simulink model "MotorModel_3"  (R2018b)
settings: Solver=VariableStepDiscrete  StartTime=0.0  StopTime=6  RelTol=1e-3  EnableMultiTasking=on
libraries: powerlib x22, powerlib_meascontrol x3, simulink x1
settings Model: Creator=LXQ  LastModifiedBy=Administrator
settings SolverCC: ZeroCrossControl=DisableAll
settings DataIOCC: LimitDataPoints=on  SaveFormat=Array
settings OptimizationCC: LifeSpan=inf
settings DebuggingCC: SolverPrmCheckMsg=warning  SFUnexpectedBacktrackingDiag=warning  SFNoUnconditionalDefaultTransitionDiag=warning  SFExecutionAtInitializationDiag=none
settings HardwareCC: ProdBitPerPointer=32  ProdBitPerSizeT=32  ProdBitPerPtrDiffT=32  ProdLargestAtomicFloat=None  ProdIntDivRoundTo=Undefined  ProdEndianess=Unspecified  ProdWordSize=32  ProdHWDeviceType=32-bit Generic
settings ModelReferenceCC: PropagateSignalLabelsOutOfModel=off
settings SFSimCC: SimUseLocalCustomCode=off
settings RTWCC: RTWUseLocalCustomCode=off
settings CodeAppCC: StateflowObjectComments=on
settings GRTTargetCC: TargetLangStandard=C89/C90 (ANSI)  GeneratePreprocessorConditionals=Disable all
settings ConfigComp: CovMetricSettings=dw  CovHtmlReporting=on  CovSaveCumulativeToWorkspaceVar=on  CovSaveSingleToWorkspaceVar=on  CovExternalEMLEnable=off  CovSFcnEnable=off
settings SimscapeCC: SimscapeNormalizeSystem=off

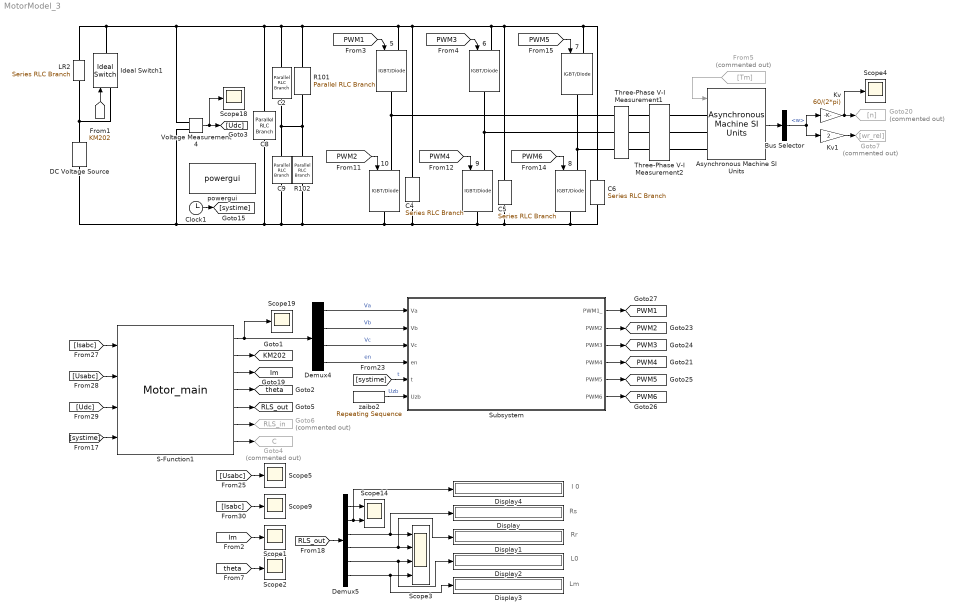
== system MotorModel_3 ==
  note: Rs
  note: Rr
  note: L0
  note: Lm
  note: I 0
  {5..10} (6 alike) : powerlib/Power Electronics/IGBT//Diode  Ron=1e-3  Rs=5000  Cs=inf  Measurements=off
      settings: SourceProductName=Simscape Electrical
  Asynchronous Machine SI Units : powerlib/Machines/Asynchronous Machine SI Units  RotorType=Squirrel-cage  PresetModel=No  MechanicalLoad=Torque Tm  ShowDetailedParameters=on  ReferenceFrame=Synchronous  Units=SI  MeasurementBus=on  NominalParameters=[41000 220 50]  Stator=[0.048 0.00031]  Rotor=[0.019 0.00031]  Cage1=[ 0.022 0.226/377]  Cage2=[ 0.022 0.226/377]  Lm=0.0133  Mechanical=[0.4 0.02187 2]  PolePairs=2  InitialConditions=[1 0 0 0 0 0 0 0]  SimulateSaturation=off  Saturation=[14.03593122, 27.81365428, 53.79336849, 72.68890987, 97.98006896, 148.6815601, 215.7428561, 302.9841135, 420.4778367 ; 230, 322, 414, 460, 506, 552, 598, 644, 690]  LoadFlowParameters=1492000  TsPowergui=0  TsBlock=-1  IterativeModel=Trapezoidal non iterative  IterativeDiscreteModel=Trapezoidal non iterative  Pmec=0
      settings: SourceProductName=Simscape Electrical
  Bus Selector : BusSelector  OutputSignals=w
  C2 : powerlib/Elements/Parallel RLC Branch  LConnTagsString=a  RConnTagsString=__new0  BranchType=C  Resistance=1  Inductance=1e-3  SetiL0=off  InitialCurrent=0  Capacitance=400e-6  Setx0=off  InitialVoltage=0  Measurements=None
      settings: SourceProductName=Simscape Electrical
  C4 : powerlib/Elements/Series RLC Branch  LConnTagsString=__new0  RConnTagsString=__new0  BranchType=C  Resistance=10  Inductance=40e-9  SetiL0=off  InitialCurrent=0  Capacitance=0.47e-6  Setx0=off  InitialVoltage=0  Measurements=None
      settings: SourceProductName=Simscape Electrical
  C5 : powerlib/Elements/Series RLC Branch  LConnTagsString=__new0  RConnTagsString=__new0  BranchType=C  Resistance=10  Inductance=40e-9  SetiL0=off  InitialCurrent=0  Capacitance=0.47e-6  Setx0=off  InitialVoltage=0  Measurements=None
      settings: SourceProductName=Simscape Electrical
  C6 : powerlib/Elements/Series RLC Branch  LConnTagsString=__new0  RConnTagsString=__new0  BranchType=C  Resistance=10  Inductance=40e-9  SetiL0=off  InitialCurrent=0  Capacitance=0.47e-6  Setx0=off  InitialVoltage=0  Measurements=None
      settings: SourceProductName=Simscape Electrical
  C8 : powerlib/Elements/Parallel RLC Branch  LConnTagsString=a  RConnTagsString=__new0  BranchType=C  Resistance=15e3  Inductance=1e-3  SetiL0=off  InitialCurrent=0  Capacitance=400e-6  Setx0=off  InitialVoltage=0  Measurements=None
      settings: SourceProductName=Simscape Electrical
  C9 : powerlib/Elements/Parallel RLC Branch  LConnTagsString=a  RConnTagsString=__new0  BranchType=C  Resistance=1  Inductance=1e-3  SetiL0=off  InitialCurrent=0  Capacitance=400e-6  Setx0=off  InitialVoltage=0  Measurements=None
      settings: SourceProductName=Simscape Electrical
  Clock1 : Clock
  DC Voltage Source : powerlib/Electrical Sources/DC Voltage Source  Amplitude=470  Measurements=None
      settings: SourceProductName=Simscape Electrical
  Demux4 : Demux
  Demux5 : Demux  Outputs=6
  Display{,1..4} (5 alike) : Display
  From5 : From  Commented=on  GotoTag=Tm
  Goto20 : Goto  Commented=on  GotoTag=n
  Goto4 : Goto  Commented=on  GotoTag=C  TagVisibility=global
  Goto6 : Goto  Commented=on  GotoTag=RLS_in  TagVisibility=global
  Goto7 : Goto  Commented=on  GotoTag=wr_rel
  Ideal Switch1 : powerlib/Power Electronics/Ideal Switch  Ron=0.0000000001  Lon=0  IC=0  Rs=1e7  Cs=inf  Measurements=off
      settings: SourceProductName=Simscape Electrical
  Kv : Gain  Gain=60/(2*pi)  SaturateOnIntegerOverflow=on  OutDataTypeStr=Inherit: Same as input  ParamDataTypeStr=Inherit: Same as input
  Kv1 : Gain  Gain=2  SaturateOnIntegerOverflow=on  OutDataTypeStr=Inherit: Same as input  ParamDataTypeStr=Inherit: Same as input
  LR2 : powerlib/Elements/Series RLC Branch  LConnTagsString=__new0  RConnTagsString=__new0  BranchType=R  Resistance=30  Inductance=200e-6  SetiL0=off  InitialCurrent=0  Capacitance=1e-6  Setx0=off  InitialVoltage=0  Measurements=None
      settings: SourceProductName=Simscape Electrical
  R101 : powerlib/Elements/Parallel RLC Branch  LConnTagsString=a  RConnTagsString=__new0  BranchType=R  Resistance=15e3  Inductance=1e-3  SetiL0=off  InitialCurrent=0  Capacitance=10800e-6  Setx0=on  InitialVoltage=110  Measurements=None
      settings: SourceProductName=Simscape Electrical
  R102 : powerlib/Elements/Parallel RLC Branch  LConnTagsString=a  RConnTagsString=__new0  BranchType=R  Resistance=15e3  Inductance=1e-3  SetiL0=off  InitialCurrent=0  Capacitance=10800e-6  Setx0=on  InitialVoltage=110  Measurements=None
      settings: SourceProductName=Simscape Electrical
  S-Function1 : S-Function  FunctionName=Motor_main  SFunctionDeploymentMode=off  EnableBusSupport=off
  Scope{1..2,4..5,9,18..19} (7 alike) : Scope
  Scope14 : Scope  NumInputPorts=2
  Scope3 : Scope  NumInputPorts=4
  Subsystem : Subsystem
  Three-Phase V-I Measurement1 : powerlib/Measurements/Three-Phase V-I Measurement  VoltageMeasurement=phase-to-phase  SetLabelV=on  LabelV=Uabc  Vpu=off  VpuLL=off  CurrentMeasurement=yes  SetLabelI=on  LabelI=Isabc  Ipu=off  Pbase=100e6  Vbase=500e3  OutputType=Complex  PhasorSimulation=off  PSBequivalent=0
      settings: SourceProductName=Simscape Electrical
  Three-Phase V-I Measurement2 : powerlib/Measurements/Three-Phase V-I Measurement  VoltageMeasurement=phase-to-phase  SetLabelV=on  LabelV=Usabc  Vpu=off  VpuLL=off  CurrentMeasurement=yes  SetLabelI=on  LabelI=Iabc  Ipu=off  Pbase=100e6  Vbase=500e3  OutputType=Complex  PhasorSimulation=off  PSBequivalent=0
      settings: SourceProductName=Simscape Electrical
  Voltage Measurement4 : powerlib/Measurements/Voltage Measurement  PhasorSimulation=off  OutputType=Complex  PSBequivalent=0
      settings: SourceProductName=Simscape Electrical
  powergui : powerlib/powergui  Priority=1  SimulationMode=Discrete  SampleTime=0.5e-6  frequency=60  Iterations=50  frequencyindice=0  Pbase=100e6  ErrMax=1e-4  UnitsV=kV  UnitsW=MW  buscounter=0  FunctionMessages=off  echomessages=off  EnableUseOfTLC=off  CurrentSourceSwitches=off  DisableSnubberDevices=off  DisableRonSwitches=off  DisableVfSwitches=off  DisplayEquations=off  SolverType=Tustin  Interpol=off  ExternalGateDelay=off  methode=off  Ts=0  x0status=blocks  SPID=off  SwTol=0  HookPort=off  RestoreLinks=warning  ResistiveCurrentMeasurement=off  Frange=[0:2:500]  Ylog=off  Xlog=on  ShowGrid=off  save=off  variable=ZData  structure=0  ZoomFFT=off  StartTime=0.0  cycles=1  DisplayStyle=1  fundamental=60  FreqAxis=off  MaxFrequency=1000  frequencyindicesteady=1  RmsSteady=1  display=off
      settings: SourceProductName=Simscape Electrical
  zaibo2 : simulink/Sources/Repeating Sequence  rep_seq_t=[0 1/10000 1/5000]  rep_seq_y=[-1 1 -1]
  tag scope: Im=global, KM202=global, PWM1=global, PWM2=global, PWM3=global, PWM4=global, PWM5=global, PWM6=global, RLS_out=global, theta=global
  wires:
  Voltage Measurement4/1 -> Scope18/1, [Udc]
  [PWM1] -> 5/1
  [PWM2] -> 10/1
  [PWM3] -> 6/1
  [PWM4] -> 9/1
  [PWM5] -> 7/1
  [PWM6] -> 8/1
  [Usabc] -> Scope5/1
  [KM202] -> Ideal Switch1/1
  Clock1/1 -> [systime]
  From5/1 -> Asynchronous Machine SI Units/1
  Asynchronous Machine SI Units/1 -> Bus Selector/1
  Bus Selector/1 -> Kv1/1, Kv/1  "<w>"
  Kv/1 -> Scope4/1, Goto20/1
  Kv1/1 -> Goto7/1
  S-Function1/1 -> Demux4/1, Scope19/1
  S-Function1/2 -> [KM202]
  S-Function1/3 -> [Im]
  [Isabc] -> S-Function1/1
  [Usabc] -> S-Function1/2
  [Udc] -> S-Function1/3
  [systime] -> S-Function1/4
  S-Function1/4 -> [theta]
  S-Function1/5 -> [RLS_out]
  S-Function1/6 -> Goto6/1
  [RLS_out] -> Demux5/1
  Demux5/2 -> Display4/1, Scope14/2
  Demux5/4 -> Scope3/2, Display1/1
  Demux5/5 -> Scope3/3, Display2/1
  Demux5/3 -> Scope3/1, Display/1
  Demux5/6 -> Scope3/4, Display3/1
  [Isabc] -> Scope9/1
  Demux5/1 -> Scope14/1
  S-Function1/7 -> Goto4/1
  [Im] -> Scope1/1
  [theta] -> Scope2/1
  Demux4/1 -> Subsystem/1(Va)  "Va"
  Demux4/2 -> Subsystem/2(Vb)  "Vb"
  Demux4/3 -> Subsystem/3(Vc)  "Vc"
  Demux4/4 -> Subsystem/4(en)  "en"
  [systime] -> Subsystem/5(t)  "t"
  zaibo2/1 -> Subsystem/6(Uzb)  "Uzb"
  Subsystem/1(PWM1_) -> [PWM1]
  Subsystem/2(PWM2) -> [PWM2]
  Subsystem/3(PWM3) -> [PWM3]
  Subsystem/4(PWM4) -> [PWM4]
  Subsystem/5(PWM5) -> [PWM5]
  Subsystem/6(PWM6) -> [PWM6]
  connections:
  9/LConn1 -- Three-Phase V-I Measurement1/LConn2 -- 6/RConn1
  LR2/RConn1 -- DC Voltage Source/RConn1 -- Ideal Switch1/LConn1
  5/RConn1 -- Three-Phase V-I Measurement1/LConn1 -- 10/LConn1
  8/LConn1 -- Three-Phase V-I Measurement1/LConn3 -- 7/RConn1
  Voltage Measurement4/LConn2 -- DC Voltage Source/LConn1 -- 10/RConn1 -- C6/RConn1 -- 8/RConn1 -- C5/RConn1 -- 9/RConn1 -- C4/RConn1 -- R102/RConn1 -- C9/RConn1 -- C8/RConn1
  Ideal Switch1/RConn1 -- Voltage Measurement4/LConn1 -- C6/LConn1 -- 7/LConn1 -- C5/LConn1 -- 6/LConn1 -- C4/LConn1 -- 5/LConn1 -- R101/LConn1 -- C2/LConn1 -- C8/LConn1 -- LR2/LConn1
  R102/LConn1 -- C9/LConn1 -- C2/RConn1 -- R101/RConn1
  Asynchronous Machine SI Units/LConn1 -- Three-Phase V-I Measurement2/RConn1
  Asynchronous Machine SI Units/LConn2 -- Three-Phase V-I Measurement2/RConn2
  Asynchronous Machine SI Units/LConn3 -- Three-Phase V-I Measurement2/RConn3
  Three-Phase V-I Measurement1/RConn2 -- Three-Phase V-I Measurement2/LConn2
  Three-Phase V-I Measurement2/LConn1 -- Three-Phase V-I Measurement1/RConn1
  Three-Phase V-I Measurement2/LConn3 -- Three-Phase V-I Measurement1/RConn3

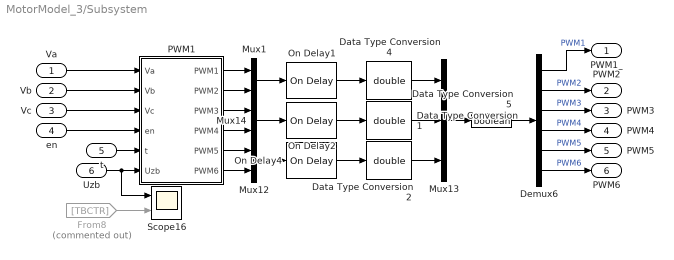
== system MotorModel_3/Subsystem ==
  Va : Inport
  Vb : Inport  Port=2
  Vc : Inport  Port=3
  en : Inport  Port=4
  t : Inport  Port=5
  Uzb : Inport  Port=6
  Data Type Conversion1 : DataTypeConversion  OutDataTypeStr=double  SaturateOnIntegerOverflow=on  RndMeth=Zero
  Data Type Conversion2 : DataTypeConversion  OutDataTypeStr=double  SaturateOnIntegerOverflow=on  RndMeth=Zero
  Data Type Conversion4 : DataTypeConversion  OutDataTypeStr=double  SaturateOnIntegerOverflow=on  RndMeth=Zero
  Data Type Conversion5 : DataTypeConversion  OutDataTypeStr=boolean
  Demux6 : Demux  Outputs=6
  From8 : From  Commented=on  GotoTag=TBCTR
  Mux1 : Mux  Inputs=2
  Mux12 : Mux  Inputs=2
  Mux13 : Mux  Inputs=3
  Mux14 : Mux  Inputs=2
  On Delay1 : powerlib_meascontrol/Logic/On Delay  DelayType=On delay  delay=1E-6  ic=0  Ts=0.1E-6
      settings: SourceProductName=Simscape Electrical
  On Delay2 : powerlib_meascontrol/Logic/On Delay  DelayType=On delay  delay=1E-6  ic=0  Ts=0.1E-6
      settings: SourceProductName=Simscape Electrical
  On Delay4 : powerlib_meascontrol/Logic/On Delay  DelayType=On delay  delay=1E-6  ic=0  Ts=0.1E-6
      settings: SourceProductName=Simscape Electrical
  PWM1 : MATLAB Function  TreatAsAtomicUnit=on
  Scope16 : Scope  NumInputPorts=2
  PWM1_ : Outport
  PWM2 : Outport  Port=2
  PWM3 : Outport  Port=3
  PWM4 : Outport  Port=4
  PWM5 : Outport  Port=5
  PWM6 : Outport  Port=6
  wires:
  Data Type Conversion4/1 -> Mux13/1
  PWM1/2(PWM2) -> Mux1/2
  On Delay1/1 -> Data Type Conversion4/1
  Mux14/1 -> On Delay2/1
  PWM1/5(PWM5) -> Mux12/1
  PWM1/3(PWM3) -> Mux14/1
  PWM1/6(PWM6) -> Mux12/2
  On Delay4/1 -> Data Type Conversion2/1
  Uzb/1 -> Scope16/1, PWM1/6(Uzb)
  PWM1/1(PWM1) -> Mux1/1
  On Delay2/1 -> Data Type Conversion1/1
  Data Type Conversion1/1 -> Mux13/2
  Mux1/1 -> On Delay1/1
  PWM1/4(PWM4) -> Mux14/2
  Mux13/1 -> Data Type Conversion5/1
  Data Type Conversion5/1 -> Demux6/1
  Data Type Conversion2/1 -> Mux13/3
  Mux12/1 -> On Delay4/1
  From8/1 -> Scope16/2
  Demux6/6 -> PWM6/1  "PWM6"
  Demux6/3 -> PWM3/1  "PWM3"
  Demux6/1 -> PWM1_/1  "PWM1"
  t/1 -> PWM1/5(t)
  Va/1 -> PWM1/1(Va)
  Demux6/5 -> PWM5/1  "PWM5"
  Demux6/2 -> PWM2/1  "PWM2"
  en/1 -> PWM1/4(en)
  Vc/1 -> PWM1/3(Vc)
  Demux6/4 -> PWM4/1  "PWM4"
  Vb/1 -> PWM1/2(Vb)

== matlab function MotorModel_3/Subsystem/PWM1 ==
  data: Va input; PWM1 output; Vb input; Vc input; en input; t input; Uzb input; PWM2 output; PWM3 output; PWM4 output; PWM5 output; PWM6 output
function [PWM1,PWM2,PWM3,PWM4,PWM5,PWM6]= PWM(Va,Vb,Vc,en,t,Uzb)

if ((t>0.1)&&(en==1))
if     (Va>Uzb)
        PWM1=1;
        PWM2=0;
else
        PWM1=0;
        PWM2=1;
end
if     (Vb>Uzb)
        PWM3=1;
        PWM4=0;
else
        PWM3=0;
        PWM4=1;
end
if     (Vc>Uzb)
        PWM5=1;
        PWM6=0;
else
        PWM5=0;
        PWM6=1;
end

else
    PWM1=0;
    PWM2=0;
    PWM3=0;
    PWM4=0;
    PWM5=0;
    PWM6=0;
end
